simulink model "ZieglerNicholsStart"  (R2015b)
settings: Solver=ode1  StartTime=0.0  StopTime=20  FixedStep=0.1  RelTol=1e-3
undefined symbols (not defined in the file or in its folder): U
settings Model: Creator=METZLER  LastModifiedBy=METZLER

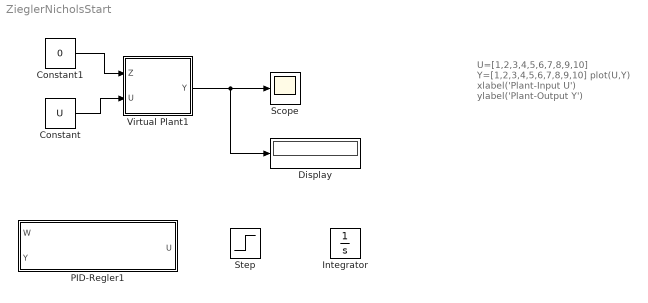
== system ZieglerNicholsStart ==
  note: U=[1,2,3,4,5,6,7,8,9,10]
      | Y=[1,2,3,4,5,6,7,8,9,10]
      | plot(U,Y)
      | xlabel('Plant-Input U')
      | ylabel('Plant-Output Y')
  Constant : Constant  Value=U
  Constant1 : Constant  Value=0
  Display : Display
  Integrator : Integrator
  PID-Regler1 : Subsystem  mask{cpc=0.5, cic=0, cdc=0, T=0.1}
      mask prompts: T "T  Time constant of real D-Part"
      mask help: A simple PID-Controller for the MOOC MSUS
      mask Display:
      | IconText='';
      | if ~strcmp(get_param(gcb,'cpc'),'0')
      |     IconText=strcat(IconText,'P');
      | end
      | if ~strcmp(get_param(gcb,'cic'),'0')
      |    IconText=strcat(IconText,'I');
      | end
      | if ~strcmp(get_param(gcb,'cdc'),'0')
      |     IconText=strcat(IconText,'D');
      | end
      | IconText=strcat(IconText,'-Controller')
      | plot(0,0)
      | plot(100,100)
      | text(25,50,IconText)
      | port_label ('output',1,'U')
      | port_label ('input',1,'W')
      | port_label ('input',2,'Y')
  Scope : Scope
  Step : Step  SampleTime=0
  Virtual Plant1 : Subsystem
  wires:
  Constant/1 -> Virtual Plant1/2(U)
  Virtual Plant1/1(Y) -> Display/1, Scope/1
  Constant1/1 -> Virtual Plant1/1(Z)

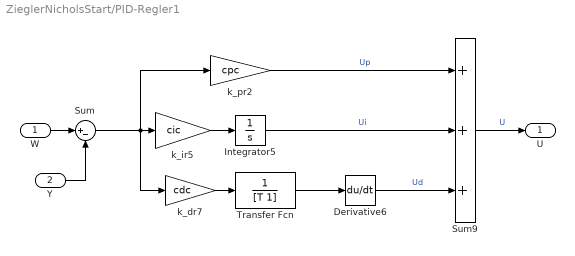
== system ZieglerNicholsStart/PID-Regler1 ==
  W : Inport
  Y : Inport  Port=2
  Derivative6 : Derivative
  Integrator5 : Integrator
  Sum : Sum  Inputs=|+-
  Sum9 : Sum  Inputs=+++
  Transfer Fcn : TransferFcn  Denominator=[T 1]
  k_dr7 : Gain  Gain=cdc
  k_ir5 : Gain  Gain=cic
  k_pr2 : Gain  Gain=cpc
  U : Outport
  wires:
  Y/1 -> Sum/2
  Sum9/1 -> U/1  "U"
  W/1 -> Sum/1
  Derivative6/1 -> Sum9/3  "Ud"
  k_pr2/1 -> Sum9/1  "Up"
  k_ir5/1 -> Integrator5/1
  Integrator5/1 -> Sum9/2  "Ui"
  Transfer Fcn/1 -> Derivative6/1
  k_dr7/1 -> Transfer Fcn/1
  Sum/1 -> k_ir5/1, k_pr2/1, k_dr7/1

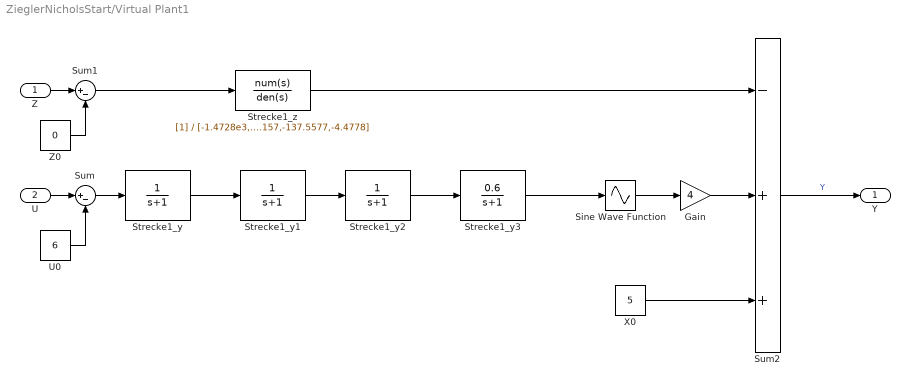
== system ZieglerNicholsStart/Virtual Plant1 ==
  Z : Inport
  U : Inport  Port=2
  Gain : Gain  Gain=4
  Sine Wave Function : Sin  TimeSource=Use external signal  SampleTime=0
  Strecke1_y : TransferFcn  Denominator=[1,1]
  Strecke1_y1 : TransferFcn  Denominator=[1,1]
  Strecke1_y2 : TransferFcn  Denominator=[1,1]
  Strecke1_y3 : TransferFcn  Numerator=[0.6]  Denominator=[1,1]
  Strecke1_z : TransferFcn  Denominator=[-1.4728e3,-534.157,-137.5577,-4.4778]
  Sum : Sum  Inputs=|+-
  Sum1 : Sum  Inputs=|+-
  Sum2 : Sum  Inputs=-++
  U0 : Constant  Value=6
  X0 : Constant  Value=5
  Z0 : Constant  Value=0
  Y : Outport
  wires:
  Sum2/1 -> Y/1  "Y"
  U/1 -> Sum/1
  Z/1 -> Sum1/1
  X0/1 -> Sum2/3
  Strecke1_z/1 -> Sum2/1
  Z0/1 -> Sum1/2
  Sum1/1 -> Strecke1_z/1
  U0/1 -> Sum/2
  Sum/1 -> Strecke1_y/1
  Strecke1_y/1 -> Strecke1_y1/1
  Strecke1_y1/1 -> Strecke1_y2/1
  Strecke1_y2/1 -> Strecke1_y3/1
  Strecke1_y3/1 -> Sine Wave Function/1
  Sine Wave Function/1 -> Gain/1
  Gain/1 -> Sum2/2
